simulink model "final_quadruped_070622_2"  (R2021a)
settings: Solver=VariableStepAuto  StartTime=0.0  StopTime=1  FixedStep=.001  RelTol=1e-3  EnableMultiTasking=on
undefined symbols (not defined in the file or in its folder): angleLFhip, convexoptimization, foot_x, foot_y, foot_z, height_plane, lower_leg_length, m_ll, m_ul, out, plane_x, plane_y, speedLFhip, torqueLFhip, torso_offset_x, torso_offset_z, torso_x, torso_y, torso_z, upper_leg_length, X, Y, Z
libraries: nesl_utility x151, sm_lib x71, Contact_Forces_Lib x16, fl_lib x4
(part 6 of 6)

== system final_quadruped_070622_2/Model/Right Leg Front /Knee/Subsystem ==
  In1 : Inport
  Derivative : Derivative
  Gain : Gain  Gain=100
  Gain1 : Gain  Gain=100
  Gain2 : Gain  Gain=100
  Integrator : Integrator
  Sum : Sum  Inputs=|+++
  Out1 : Outport
  wires:
  Sum/1 -> Out1/1
  Gain2/1 -> Sum/3
  In1/1 -> Derivative/1, Gain2/1, Integrator/1
  Derivative/1 -> Gain/1
  Gain/1 -> Sum/1
  Integrator/1 -> Gain1/1
  Gain1/1 -> Sum/2

== matlab function final_quadruped_070622_2/Model/Left Leg Front/Subsystem/MATLAB Function ==
  data: eb1g output; eb2g output; eb3g output; qhb input; qab input; Qquat input; qkb input; ab1g output; ab2g output; cmb1g output; cmb2g output; cmb3g output; Qd3g output
function [eb1g,eb2g,eb3g,ab1g,ab2g,cmb1g,cmb2g,cmb3g,Qd3g] = fcn(qhb,qab,Qquat,qkb)
eb1g = zeros([3 1], 'double');
eb2g = zeros([3 1], 'double');
eb3g = zeros([3 1], 'double');
ab1g = zeros([3 1], 'double');
ab2g = zeros([3 1], 'double');
cmb1g = zeros([3 1], 'double');
cmb2g = zeros([3 1], 'double');
cmb3g = zeros([3 1], 'double');
Qd3g = zeros([3 3], 'double');
coder.extrinsic('lfval_mex');
[eb1g,eb2g,eb3g,ab1g,ab2g,cmb1g,cmb2g,cmb3g,Qd3g] = lfval_mex(qhb,qab,Qquat,qkb);
end

== matlab function final_quadruped_070622_2/Model/Right Leg Back/Subsystem/MATLAB Function ==
  data: ec1g output; ec2g output; ec3g output; qhc input; qac input; Qquat input; qkc input; ac1g output; ac2g output; cmc1g output; cmc2g output; cmc3g output; Qd3g output
function [ec1g,ec2g,ec3g,ac1g,ac2g,cmc1g,cmc2g,cmc3g,Qd3g] = fcn(qhc,qac,Qquat,qkc)
ec1g = zeros([3 1], 'double');
ec2g = zeros([3 1], 'double');
ec3g = zeros([3 1], 'double');
ac1g = zeros([3 1], 'double');
ac2g = zeros([3 1], 'double');
cmc1g = zeros([3 1], 'double');
cmc2g = zeros([3 1], 'double');
cmc3g = zeros([3 1], 'double');
Qd3g = zeros([3 3], 'double');
coder.extrinsic('rbval_mex');
[ec1g,ec2g,ec3g,ac1g,ac2g,cmc1g,cmc2g,cmc3g,Qd3g] = rbval_mex(qhc,qac,Qquat,qkc);
end

== matlab function final_quadruped_070622_2/Model/Left LegBack/Subsystem/MATLAB Function ==
  data: ed1g output; ed2g output; ed3g output; qhd input; qad input; Qquat input; qkd input; ad1g output; ad2g output; cmd1g output; cmd2g output; cmd3g output; Qd3g output
function [ed1g,ed2g,ed3g,ad1g,ad2g,cmd1g,cmd2g,cmd3g,Qd3g] = fcn(qhd,qad,Qquat, qkd)
ed1g = zeros([3 1], 'double');
ed2g = zeros([3 1], 'double');
ed3g = zeros([3 1], 'double');
ad1g = zeros([3 1], 'double');
ad2g = zeros([3 1], 'double');
cmd1g = zeros([3 1], 'double');
cmd2g = zeros([3 1], 'double');
cmd3g = zeros([3 1], 'double');
Qd3g = zeros([3 3], 'double');
coder.extrinsic('lbval_mex');
[ed1g,ed2g,ed3g,ad1g,ad2g,cmd1g,cmd2g,cmd3g,Qd3g] = lbval_mex(qhd,qad,Qquat, qkd);
end

== matlab function final_quadruped_070622_2/Model/MATLAB Function4 ==
  data: hLF input; hRB input; hLB input; h_dotLF input; hRF input; h_dotRF input; tddRF output; v_torso input; tddLF output; tddRB output; tddLB output; h output; h_dot output; h_dotRB input; h_dotLB input; theta_d_des output; M output; V input
function [tddRF,tddLF,tddRB,tddLB,h,h_dot,theta_d_des,M] = fcn(hLF, hRB, hLB, h_dotLF, hRF,h_dotRF, v_torso, h_dotRB, h_dotLB, V)
% tddRF = zeros([3 1], 'double');
% tddLF = zeros([3 1], 'double');
% tddRB = zeros([3 1], 'double');
% tddLB = zeros([3 1], 'double');
% h = zeros([3 12], 'double');
% h_dot = zeros([3 12], 'double');
% theta_d_des = zeros([12 1], 'double');
% M = zeros(1, 'double');
% coder.extrinsic('theta_d_des_mex');
% [tddRF,tddLF,tddRB,tddLB,h,h_dot,theta_d_des,M] = theta_d_des_mex(hLF, hRB, hLB, h_dotLF, hRF,h_dotRF, v_torso, h_dotRB, h_dotLB);
lower_leg_length = 10;
upper_leg_length = 10;
density = 1000;
foot_density=2000;
leg_radius = 0.75;
foot_x = 8;
foot_y = 6;
foot_z = 1;
torso_y = 16;
torso_x = 25;
torso_z = 10;
m_ul=density*leg_radius*leg_radius*upper_leg_length*3.141592653589*0.01*0.01*0.01;
m_ll=density*leg_radius*leg_radius*lower_leg_length*3.141592653589*0.01*0.01*0.01;
m_foot=foot_density*foot_x*foot_y*foot_z*0.000001;
m_torso=density*torso_x*torso_y*torso_z*0.000001;
M=m_torso+(4*(m_ul+m_ll+m_foot));
%%
h=[hRF hLF hRB hLB];
% A=transpose(h)*h;
% [V,D]=eig(A);
% VR=real(V);
% %coder.extrinsic('chooseJVoptimize');
h_dot=[h_dotRF h_dotLF h_dotRB h_dotLB];
% %theta_d_des=chooseJVoptimize(h,h_dot,v_torso, M);
% % 
% theta_d_des=M*(-pinv(h)*v_torso)+VR(:,1);
% % % theta_d_des=zeros(12,1);
% % x=zeros(12,9);
% % y=zeros(12,9);
% % ynorm=zeros(9,1);
% % for i=1:9
% %     x(:,i)=M*(-pinv(h)*v_torso)+real(V(:,i));
% %     y(:,i)=pinv(h)*(-h_dot*x(:,i));
% %     ynorm(i)=norm(y(:,i));
% % end
% % ynormmin=min(ynorm);
% % 
% % for i=1:9
% %     if ynorm(i)==ynormmin
% %         theta_d_des=x(:,i);
% %     end
% % end
 w=zeros(9,1);
% %w = [0.01;0.03;0.05;0.01;0.03;0.04;0.02;0.005;0.6];
% Va=VR(:,1:9);
% %tddfun = @(w) norm(-pinv(h)*h_dot*M*(-pinv(h)*v_torso+Va*w));
% tddfun = @(w) norm(-pinv(h)*h_dot*(Va*w));
% A = Va;
% b = 0.5*ones(12,1);
% %Aeq = [transpose(x(2:10))*x(2:10)*ones(12,1),(x(1)*eye(12,12)-pinv(Reh)*Rehdot)*Va];
% Aeq = [];
% 
% beq = [];
% lb = [];
% ub =[];
% %nonlcon =norm(w)-1;
% w0 = [0.01;0.03;0.05;0.01;0.03;0.04;0.05;0.02;0.06];
% options=optimoptions('fmincon', 'Algorithm', 'sqp');
%  w= fmincon(tddfun,w0,A,b,[],[],[],[],[],options);
%theta_d_des=Va*w;
VR=real(V);
Va=VR(:,1:9);
% theta_d_des=M*(-pinv(h)*v_torso)+VR(:,1);
% Va=VR(:,1:9);
% 
% 
% w1=1;w2=2;w3=3;w4=4;w5=5;w6=6;w7=7;w8=8;w9=9;
% 
% cvx_begin
%     variables w1 w2 w3 w4 w5 w6 w7 w8 w9
%     minimize(norm(-pinv(h)*h_dot*(Va*[w1;w2;w3;w4;w5;w6;w7;w8;w9])));
%     subject to
%         Va*[w1;w2;w3;w4;w5;w6;w7;w8;w9] < 0.5*ones(12,1);
% cvx_end
% 
% w=[w1;w2;w3;w4;w5;w6;w7;w8;w9];
% theta_d_des=Va*w;

% [w]=convexoptimization(VR,h,h_dot);
 theta_d_des=Va*w;
 
tddRF_hip=theta_d_des(1);
tddRF_knee=theta_d_des(2);
tddRF_ankle=theta_d_des(3);
tddLF_hip=theta_d_des(4);
tddLF_knee=theta_d_des(5);
tddLF_ankle=theta_d_des(6);
tddRB_hip=theta_d_des(7);
tddRB_knee=theta_d_des(8);
tddRB_ankle=theta_d_des(9);
tddLB_hip=theta_d_des(10);
tddLB_knee=theta_d_des(11);
tddLB_ankle=theta_d_des(12);

tddRF=[tddRF_hip tddRF_knee tddRF_ankle];
tddLF=[tddLF_hip tddLF_knee tddLF_ankle];
tddRB=[tddRB_hip tddRB_knee tddRB_ankle];
tddLB=[tddLB_hip tddLB_knee tddLB_ankle];
end

== matlab function final_quadruped_070622_2/Model/Right Leg Front /Subsystem/MATLAB Function1 ==
  data: ea10g input; ea20g input; aa10g input; cma2 input; cma1 input; cma3 input; ea30g input; aa20g input; hRF output; rhoRF output
function [hRF,rhoRF] = fcn(ea10g, ea20g, aa10g, cma2, cma1, cma3, ea30g, aa20g)
hRF = zeros([3 3], 'double');
rhoRF = zeros([3 3 3], 'double');
coder.extrinsic('hrfrhorf_mex');
[hRF,rhoRF] = hrfrhorf_mex(ea10g, ea20g, aa10g, cma2, cma1, cma3, ea30g, aa20g);
end

== matlab function final_quadruped_070622_2/Model/Left Leg Front/Subsystem/MATLAB Function1 ==
  data: eb10g input; eb20g input; ab10g input; cmb2 input; cmb1 input; cmb3 input; eb30g input; hLF output; ab20g input; rhoLF output
function [hLF,rhoLF] = fcn(eb10g, eb20g, ab10g, cmb2, cmb1, cmb3, eb30g, ab20g)
hLF = zeros([3 3], 'double');
rhoLF = zeros([3 3 3], 'double');
coder.extrinsic('hlfrholf_mex');
[hLF,rhoLF] = hlfrholf_mex(eb10g, eb20g, ab10g, cmb2, cmb1, cmb3, eb30g, ab20g);
end

== matlab function final_quadruped_070622_2/Model/Right Leg Back/Subsystem/MATLAB Function1 ==
  data: ec10g input; ec20g input; ac10g input; cmc2 input; cmc1 input; cmc3 input; ec30g input; ac20g input; hRB output; rhoRB output
function [hRB,rhoRB] = fcn(ec10g, ec20g, ac10g, cmc2, cmc1, cmc3, ec30g, ac20g)
hRB = zeros([3 3], 'double');
rhoRB = zeros([3 3 3], 'double');
coder.extrinsic('hrbrhorb_mex');
[hRB,rhoRB] = hrbrhorb_mex(ec10g, ec20g, ac10g, cmc2, cmc1, cmc3, ec30g, ac20g);
end

== matlab function final_quadruped_070622_2/Model/Left LegBack/Subsystem/MATLAB Function1 ==
  data: ed10g input; ed20g input; ad10g input; cmd2 input; cmd1 input; cmd3 input; ed30g input; ad20g input; hLB output; rhoLB output
function [hLB,rhoLB] = fcn(ed10g, ed20g, ad10g, cmd2, cmd1, cmd3, ed30g, ad20g)
hLB = zeros([3 3], 'double');
rhoLB = zeros([3 3 3], 'double');
coder.extrinsic('hlbrholb_mex');
[hLB,rhoLB] = hlbrholb_mex(ed10g, ed20g, ad10g, cmd2, cmd1, cmd3, ed30g, ad20g);
end

== matlab function final_quadruped_070622_2/MATLAB Function ==
  data: vx input; v_torso output; vy input; vz input
function v_torso = fcn(vx, vy, vz)
v_torso=[vx; vy; vz];
end

== matlab function final_quadruped_070622_2/Model/Right Leg Front /MATLAB Function2 ==
  data: tddRF input; tddRF_hip output; tddRF_knee output; tddRF_ankle output
function [tddRF_hip, tddRF_knee, tddRF_ankle] = fcn(tddRF)
tddRF_hip = zeros(1, 'double');
tddRF_knee = zeros(1, 'double');
tddRF_ankle = zeros(1, 'double');
coder.extrinsic('rf2_mex');
[tddRF_hip, tddRF_knee, tddRF_ankle] = rf2_mex(tddRF);
end

== matlab function final_quadruped_070622_2/Subsystem/MATLAB Function1 ==
  data: vx input; vy input; v output; vz input; ax input; ay input; az input; a output
function [v,a] = fcn(vx,vy,vz,ax,ay,az)
v=[vx;vy;vz];
a=[ax;ay;az];
end

== matlab function final_quadruped_070622_2/Model/Left Leg Front/MATLAB Function2 ==
  data: tddLF input; tddLF_hip output; tddLF_knee output; tddLF_ankle output
function [tddLF_hip, tddLF_knee, tddLF_ankle] = fcn(tddLF)
tddLF_hip = zeros(1, 'double');
tddLF_knee = zeros(1, 'double');
tddLF_ankle = zeros(1, 'double');
coder.extrinsic('lf2_mex');
[tddLF_hip, tddLF_knee, tddLF_ankle] = lf2_mex(tddLF);
end

== matlab function final_quadruped_070622_2/Model/Right Leg Back/MATLAB Function2 ==
  data: tddRB input; tddRB_hip output; tddRB_knee output; tddRB_ankle output
function [tddRB_hip, tddRB_knee, tddRB_ankle] = fcn(tddRB)
tddRB_hip=zeros(1,'double');
tddRB_knee=zeros(1,'double');
tddRB_ankle=zeros(1,'double');
coder.extrinsic('rb2_mex');
[tddRB_hip, tddRB_knee, tddRB_ankle] = rb2_mex(tddRB);
end

== matlab function final_quadruped_070622_2/Model/Left LegBack/MATLAB Function2 ==
  data: tddLB input; tddLB_hip output; tddLB_knee output; tddLB_ankle output
function [tddLB_hip, tddLB_knee, tddLB_ankle] = fcn(tddLB)
tddLB_hip=zeros(1,'double');
tddLB_knee=zeros(1,'double');
tddLB_ankle=zeros(1,'double');
coder.extrinsic('lb2_mex');
[tddLB_hip, tddLB_knee, tddLB_ankle] = lb2_mex(tddLB);
end

== matlab function final_quadruped_070622_2/Subsystem/MATLAB Function4 ==
  data: vx input; vy input; v output; vz input; ax input; ay input; az input; a output
function [v,a] = fcn(vx,vy,vz,ax,ay,az)
v=[vx;vy;vz];
a=[ax;ay;az];
end

== matlab function final_quadruped_070622_2/Subsystem/MATLAB Function5 ==
  data: vx input; vy input; v output; vz input; ax input; ay input; az input; a output
function [v,a] = fcn(vx,vy,vz,ax,ay,az)
v=[vx;vy;vz];
a=[ax;ay;az];
end

== matlab function final_quadruped_070622_2/Subsystem/MATLAB Function6 ==
  data: vx input; vy input; v output; vz input; ax input; ay input; az input; a output
function [v,a] = fcn(vx,vy,vz,ax,ay,az)
v=[vx;vy;vz];
a=[ax;ay;az];
end

== matlab function final_quadruped_070622_2/Subsystem/MATLAB Function7 ==
  data: vx input; vy input; v output; vz input; ax input; ay input; az input; a output
function [v,a] = fcn(vx,vy,vz,ax,ay,az)
v=[vx;vy;vz];
a=[ax;ay;az];
end

== matlab function final_quadruped_070622_2/Subsystem/MATLAB Function8 ==
  data: vx input; vy input; v output; vz input; ax input; ay input; az input; a output
function [v,a] = fcn(vx,vy,vz,ax,ay,az)
v=[vx;vy;vz];
a=[ax;ay;az];
end

== matlab function final_quadruped_070622_2/Subsystem/MATLAB Function9 ==
  data: vx input; vy input; v output; vz input; ax input; ay input; az input; a output
function [v,a] = fcn(vx,vy,vz,ax,ay,az)
v=[vx;vy;vz];
a=[ax;ay;az];
end

== matlab function final_quadruped_070622_2/Subsystem/MATLAB Function10 ==
  data: vx input; vy input; v output; vz input; ax input; ay input; az input; a output
function [v,a] = fcn(vx,vy,vz,ax,ay,az)
v=[vx;vy;vz];
a=[ax;ay;az];
end

== matlab function final_quadruped_070622_2/Subsystem/MATLAB Function11 ==
  data: vx input; vy input; v output; vz input; ax input; ay input; az input; a output
function [v,a] = fcn(vx,vy,vz,ax,ay,az)
v=[vx;vy;vz];
a=[ax;ay;az];
end

== matlab function final_quadruped_070622_2/Subsystem/MATLAB Function13 ==
  data: vulRF input; vllRF input; Mvcm output; vfRF input; vulLF input; vllLF input; vfLF input; vulRB input; vllRB input; vfRB input; vulLB input; vllLB input; vfLB input; v_torso input; vlinks output; vcm output
function [Mvcm,vlinks,vcm] = fcn(vulRF,vllRF,vfRF,vulLF,vllLF,vfLF,vulRB,vllRB,vfRB,vulLB,vllLB,vfLB,v_torso)
%%
lower_leg_length = 10;
upper_leg_length = 10;
density = 1000;
foot_density=2000;
leg_radius = 0.75;
foot_x = 8;
foot_y = 6;
foot_z = 1;
torso_y = 16;
torso_x = 25;
torso_z = 10;
m_ul=density*leg_radius*leg_radius*upper_leg_length*3.141592653589*0.01*0.01*0.01;
m_ll=density*leg_radius*leg_radius*lower_leg_length*3.141592653589*0.01*0.01*0.01;
m_foot=foot_density*foot_x*foot_y*foot_z*0.000001;
m_torso=density*torso_x*torso_y*torso_z*0.000001;
M=m_torso+4*(m_ul+m_ll+m_foot);
%%
Mvcm=m_torso*v_torso+(m_ul*vulRF+m_ll*vllRF+m_foot*vfRF)+(m_ul*vulLF+m_ll*vllLF+m_foot*vfLF)+(m_ul*vulRB+m_ll*vllRB+m_foot*vfRB)+(m_ul*vulLB+m_ll*vllLB+m_foot*vfLB);
vlinks=[vulRF vllRF vfRF vulLF vllLF vfLF vulRB vllRB vfRB vulLB vllLB vfLB];
vcm=Mvcm/M;
end

== matlab function final_quadruped_070622_2/Subsystem/MATLAB Function12 ==
  data: vx input; vy input; v output; vz input; ax input; ay input; az input; a output
function [v,a] = fcn(vx,vy,vz,ax,ay,az)
v=[vx;vy;vz];
a=[ax;ay;az];
end

== matlab function final_quadruped_070622_2/Subsystem/MATLAB Function14 ==
  data: vx input; vy input; v output; vz input; ax input; ay input; az input; a output
function [v,a] = fcn(vx,vy,vz,ax,ay,az)
v=[vx;vy;vz];
a=[ax;ay;az];
end

== matlab function final_quadruped_070622_2/Model/Right Leg Front /MATLAB Function ==
  data: ankle input; knee input; tdRF output; hip input
function tdRF= fcn(ankle, knee, hip)
tdRF = zeros([3 1], 'double');
coder.extrinsic('rf3_mex');
tdRF=rf3_mex(ankle, knee, hip);
end

== matlab function final_quadruped_070622_2/Model/Left Leg Front/MATLAB Function ==
  data: ankle input; knee input; tdRF output; hip input
function tdRF= fcn(ankle, knee, hip)
tdRF = zeros([3 1], 'double');
coder.extrinsic('lf3_mex');
tdRF= lf3_mex(ankle, knee, hip);
end

== matlab function final_quadruped_070622_2/Model/Right Leg Back/MATLAB Function ==
  data: ankle input; knee input; tdRB output; hip input
function tdRB= fcn(ankle, knee, hip)
tdRB=zeros([3 1],'double');
coder.extrinsic('rb3_mex');
tdRB= rb3_mex(ankle, knee, hip);
end

== matlab function final_quadruped_070622_2/Model/Left LegBack/MATLAB Function ==
  data: ankle input; knee input; tdLB output; hip input
function tdLB= fcn(ankle, knee, hip)
tdLB=zeros([3 1],'double');
coder.extrinsic('lb3_mex');
tdLB= lb3_mex(ankle, knee, hip);
end

== matlab function final_quadruped_070622_2/Model/MATLAB Function ==
  data: tdRF input; td output; tdLF input; tdRB input; tdLB input; t2dRF input; t2dLF input; t2dRB input; t2dLB input; t2d output
function [td,t2d] = fcn(tdRF,tdLF,tdRB,tdLB,t2dRF,t2dLF,t2dRB,t2dLB)
td = zeros([12 1], 'double');
t2d = zeros([12 1], 'double');
coder.extrinsic('acttheta_mex');
[td,t2d] = acttheta_mex(tdRF,tdLF,tdRB,tdLB,t2dRF,t2dLF,t2dRB,t2dLB);
end

== matlab function final_quadruped_070622_2/Model/MATLAB Function1 ==
  data: h input; h_dot input; ht2d output; td input; t2d input; h_dottd output; htd output; theta_d_des input; theta_2d_des input; ht2ddes output; hdtddes output
function [ht2d,h_dottd,htd,ht2ddes,hdtddes] = fcn(h,h_dot, td, t2d,theta_d_des,theta_2d_des)
ht2d = zeros([3 1], 'double');
h_dottd = zeros([3 1], 'double');
htd = zeros([3 1], 'double');
ht2ddes = zeros([3 1], 'double');
hdtddes = zeros([3 1], 'double');
coder.extrinsic('findh_mex');
[ht2d,h_dottd,htd,ht2ddes,hdtddes] = findh_mex(h,h_dot, td, t2d,theta_d_des,theta_2d_des);
end

== matlab function final_quadruped_070622_2/MATLAB Function1 ==
  data: Mvcm input; error output; ht2d input; h_dottd input; a_torso input; v_torso input; f input; Macm input; htd input; ht2ddes input; hdtddes input
function error = fcn(Mvcm,ht2d,h_dottd,a_torso, v_torso, f,Macm,htd, ht2ddes, hdtddes)
%%
lower_leg_length = 10;
upper_leg_length = 10;
density = 1000;
foot_density=2000;
leg_radius = 0.75;
foot_x = 8;
foot_y = 6;
foot_z = 1;
torso_y = 16;
torso_x = 25;
torso_z = 10;
m_ul=density*leg_radius*leg_radius*upper_leg_length*3.141592653589*0.01*0.01*0.01;
m_ll=density*leg_radius*leg_radius*lower_leg_length*3.141592653589*0.01*0.01*0.01;
m_foot=foot_density*foot_x*foot_y*foot_z*0.000001;
m_torso=density*torso_x*torso_y*torso_z*0.000001;
M=m_torso+(4*(m_ul+m_ll+m_foot));
g=[0; 0; -9.80067];
%%
error1=htd+M*v_torso-Mvcm;
error2=ht2d+h_dottd+M*a_torso-M*g-f-Macm;
error=ht2ddes+hdtddes+M*a_torso-M*g-f-Macm;
end

== matlab function final_quadruped_070622_2/Model/Right Leg Front /Subsystem/MATLAB Function2 ==
  data: h_dotRF output; ea_dg1 input; ea1g input; ea2g input; ea3g input; ea_dg2 input; ea_dg3 input; rho_dotRF input; rhoRF input
function h_dotRF = fcn(  ea_dg1,ea1g, ea2g, ea3g, ea_dg2, ea_dg3, rho_dotRF, rhoRF)
h_dotRF = zeros([3 3], 'double');
coder.extrinsic('hdotrf_mex');
h_dotRF = hdotrf_mex(ea_dg1,ea1g, ea2g, ea3g, ea_dg2, ea_dg3, rho_dotRF, rhoRF);
end

== matlab function final_quadruped_070622_2/Model/Left Leg Front/Subsystem/MATLAB Function2 ==
  data: h_dotLF output; eb_dg1 input; eb1g input; eb2g input; eb3g input; eb_dg2 input; eb_dg3 input; rho_dotLF input; rhoLF input
function h_dotLF = fcn( eb_dg1,eb1g, eb2g, eb3g, eb_dg2, eb_dg3, rho_dotLF, rhoLF)
h_dotLF = zeros([3 3], 'double');
coder.extrinsic('hdotlf_mex');
h_dotLF = hdotlf_mex( eb_dg1,eb1g, eb2g, eb3g, eb_dg2, eb_dg3, rho_dotLF, rhoLF);

end

== matlab function final_quadruped_070622_2/Model/Right Leg Front /Subsystem/MATLAB Function4 ==
  data: ea1g input; ea2g input; aa1g input; aa2g input; ea3g input; vlinks input; w_torso input; ea_dg1 output; td1 input; v_torso input; ea_dg2 output; td2 input; td3 input; ea_dg3 output; rho_dotRF output
function [ea_dg1,ea_dg2,ea_dg3,rho_dotRF] = fcn(ea1g,ea2g,aa1g,aa2g, ea3g, vlinks, w_torso, td1, v_torso, td2, td3)
ea_dg1 = zeros([3 1], 'double');
ea_dg2 = zeros([3 1], 'double');
ea_dg3 = zeros([3 1], 'double');
rho_dotRF = zeros([3 3 3], 'double');
coder.extrinsic('rfval1_mex');
[ea_dg1,ea_dg2,ea_dg3,rho_dotRF] = rfval1_mex(ea1g,ea2g,aa1g,aa2g, ea3g, vlinks, w_torso, td1, v_torso, td2, td3);

end

== matlab function final_quadruped_070622_2/Model/Left Leg Front/Subsystem/MATLAB Function4 ==
  data: eb1g input; eb2g input; ab1g input; ab2g input; eb3g input; vlinks input; w_torso input; eb_dg1 output; td1 input; v_torso input; eb_dg2 output; td2 input; td3 input; eb_dg3 output; rho_dotLF output
function [eb_dg1,eb_dg2,eb_dg3,rho_dotLF] = fcn(eb1g,eb2g,ab1g,ab2g, eb3g, vlinks, w_torso, td1, v_torso, td2, td3)
eb_dg1 = zeros([3 1], 'double');
eb_dg2 = zeros([3 1], 'double');
eb_dg3 = zeros([3 1], 'double');
rho_dotLF = zeros([3 3 3], 'double');
coder.extrinsic('lfval1_mex');
[eb_dg1,eb_dg2,eb_dg3,rho_dotLF] = lfval1_mex(eb1g,eb2g,ab1g,ab2g, eb3g, vlinks, w_torso, td1, v_torso, td2, td3);

end

== matlab function final_quadruped_070622_2/Model/Right Leg Back/Subsystem/MATLAB Function2 ==
  data: h_dotRB output; ec_dg1 input; ec1g input; ec2g input; ec3g input; ec_dg2 input; ec_dg3 input; rho_dotRB input; rhoRB input
function h_dotRB = fcn( ec_dg1,ec1g, ec2g, ec3g, ec_dg2, ec_dg3, rho_dotRB, rhoRB)
h_dotRB = zeros([3 3], 'double');
coder.extrinsic('hdotrb_mex');
h_dotRB = hdotrb_mex( ec_dg1,ec1g, ec2g, ec3g, ec_dg2, ec_dg3, rho_dotRB, rhoRB);
end

== matlab function final_quadruped_070622_2/Model/Right Leg Back/Subsystem/MATLAB Function4 ==
  data: ec1g input; ec2g input; ac1g input; ac2g input; ec3g input; vlinks input; w_torso input; ec_dg1 output; td1 input; v_torso input; ec_dg2 output; td2 input; td3 input; ec_dg3 output; rho_dotRB output
function [ec_dg1,ec_dg2,ec_dg3,rho_dotRB] = fcn(ec1g,ec2g,ac1g,ac2g, ec3g, vlinks, w_torso, td1, v_torso, td2, td3)
ec_dg1 = zeros([3 1], 'double');
ec_dg2 = zeros([3 1], 'double');
ec_dg3 = zeros([3 1], 'double');
rho_dotRB = zeros([3 3 3], 'double');
coder.extrinsic('rbval1_mex');
[ec_dg1,ec_dg2,ec_dg3,rho_dotRB] = rbval1_mex(ec1g,ec2g,ac1g,ac2g, ec3g, vlinks, w_torso, td1, v_torso, td2, td3);

end

== matlab function final_quadruped_070622_2/Subsystem/MATLAB Function2 ==
  data: vx input; vy input; v output; vz input; ax input; ay input; az input; a output
function [v,a] = fcn(vx,vy,vz,ax,ay,az)
v=[vx;vy;vz];
a=[ax;ay;az];
end

== matlab function final_quadruped_070622_2/Model/Left LegBack/Subsystem/MATLAB Function2 ==
  data: h_dotLB output; ed_dg1 input; ed1g input; ed2g input; ed3g input; ed_dg2 input; ed_dg3 input; rho_dotLB input; rhoLB input
function h_dotLB = fcn( ed_dg1,ed1g, ed2g, ed3g, ed_dg2, ed_dg3, rho_dotLB, rhoLB)
h_dotLB = zeros([3 3], 'double');
coder.extrinsic('hdotlb_mex');
h_dotLB = hdotlb_mex( ed_dg1,ed1g, ed2g, ed3g, ed_dg2, ed_dg3, rho_dotLB, rhoLB);
end

== matlab function final_quadruped_070622_2/Model/Left LegBack/Subsystem/MATLAB Function4 ==
  data: ed1g input; ed2g input; ad1g input; ad2g input; ed3g input; vlinks input; w_torso input; ed_dg1 output; td1 input; v_torso input; ed_dg2 output; td2 input; td3 input; ed_dg3 output; rho_dotLB output
function [ed_dg1,ed_dg2,ed_dg3,rho_dotLB] = fcn(ed1g,ed2g,ad1g,ad2g, ed3g, vlinks, w_torso, td1, v_torso, td2, td3)
ed_dg1 = zeros([3 1], 'double');
ed_dg2 = zeros([3 1], 'double');
ed_dg3 = zeros([3 1], 'double');
rho_dotLB = zeros([3 3 3], 'double');
coder.extrinsic('lbval1_mex');
[ed_dg1,ed_dg2,ed_dg3,rho_dotLB] = lbval1_mex(ed1g,ed2g,ad1g,ad2g, ed3g, vlinks, w_torso, td1, v_torso, td2, td3);
end

== matlab function final_quadruped_070622_2/Model/Left Leg Front/MATLAB Function1 ==
  data: ankle input; knee input; t2dLF output; hip input
function t2dLF= fcn(ankle, knee, hip)
t2dLF = zeros([3 1], 'double');
coder.extrinsic('lf4_mex');
t2dLF= lf4_mex(ankle, knee, hip);
end

== matlab function final_quadruped_070622_2/Model/Right Leg Front /MATLAB Function1 ==
  data: ankle input; knee input; t2dRF output; hip input
function t2dRF= fcn(ankle, knee, hip)
t2dRF = zeros([3 1], 'double');
coder.extrinsic('rf4_mex');
t2dRF= rf4_mex(ankle, knee, hip);
end

== matlab function final_quadruped_070622_2/MATLAB Function2 ==
  data: ax input; a_torso output; ay input; az input
function a_torso = fcn(ax, ay, az)
a_torso=[ax; ay; az];
end

== matlab function final_quadruped_070622_2/Model/Left Leg Front/Contact Forces /MATLAB Function ==
  data: n1 input; NLF output; n2 input; n4 input; n3 input; f1 input; f2 input; f3 input; f4 input; FLF output; Qd3g input
function [NLF,FLF] = fcn(n1,n2,n4,n3,f1,f2,f3,f4, Qd3g)
Qds3=[1 0 0;
      0 cos(90) -sin(90);
      0 sin(90) cos(90)];
% mu_s = 0.8;
% alpha=atan(mu_s);
% NRF=n1+n2+n3+n4;
% FRFca=f1*cos(alpha)+f2*cos(alpha)+f3*cos(alpha)+f4*cos(alpha);
% FRFsa=f1*sin(alpha)+f2*sin(alpha)+f3*sin(alpha)+f4*sin(alpha);
NLF=n1+n2+n3+n4;
FLF=f1+f2+f3+f4;
FLF=Qds3*Qd3g*FLF;
end

== matlab function final_quadruped_070622_2/Model/MATLAB Function2 ==
  data: theta_d_des input; theta_2d_des output; h_dot input; h input; a_torso input; M input; f input
function theta_2d_des = fcn(theta_d_des, h_dot, h, a_torso, M, f)
 theta_2d_des = zeros([12 1], 'double');
 coder.extrinsic('theta_2d_des_mex'); 
 theta_2d_des=theta_2d_des_mex(theta_d_des, h_dot, h, a_torso, M, f);
%theta_2d_des=zeros([12 1],'double');
end

== matlab function final_quadruped_070622_2/Model/Right Leg Front /Contact Forces /MATLAB Function ==
  data: n1 input; NRF output; n2 input; n4 input; n3 input; f1 input; f2 input; f3 input; f4 input; FRF output; Qd3g input
function [NRF,FRF] = fcn(n1,n2,n4,n3,f1,f2,f3,f4, Qd3g)
% mu_s = 0.8;
% alpha=atan(mu_s);
% NRF=n1+n2+n3+n4;
% FRFca=f1*cos(alpha)+f2*cos(alpha)+f3*cos(alpha)+f4*cos(alpha);
% FRFsa=f1*sin(alpha)+f2*sin(alpha)+f3*sin(alpha)+f4*sin(alpha);
Qds3=[1 0 0;
      0 cos(90) -sin(90);
      0 sin(90) cos(90)];
NRF=n1+n2+n3+n4;
FRFl=f1+f2+f3+f4;
FRF=Qds3*Qd3g*FRFl;
end

== matlab function final_quadruped_070622_2/Model/Right Leg Back/Contact Forces /MATLAB Function ==
  data: n1 input; NRB output; n2 input; n4 input; n3 input; f1 input; f2 input; f3 input; f4 input; FRB output; Qd3g input
function [NRB,FRB] = fcn(n1,n2,n4,n3,f1,f2,f3,f4,Qd3g)
Qds3=[1 0 0;
      0 cos(90) -sin(90);
      0 sin(90) cos(90)];
% mu_s = 0.8;
% alpha=atan(mu_s);
% NRF=n1+n2+n3+n4;
% FRFca=f1*cos(alpha)+f2*cos(alpha)+f3*cos(alpha)+f4*cos(alpha);
% FRFsa=f1*sin(alpha)+f2*sin(alpha)+f3*sin(alpha)+f4*sin(alpha);
NRB=n1+n2+n3+n4;
FRB=f1+f2+f3+f4;
FRB=Qds3*Qd3g*FRB;
end

== matlab function final_quadruped_070622_2/Subsystem/MATLAB Function3 ==
  data: vx input; vy input; v output; vz input; ax input; ay input; az input; a output
function [v,a] = fcn(vx,vy,vz,ax,ay,az)
v=[vx;vy;vz];
a=[ax;ay;az];
end

== matlab function final_quadruped_070622_2/Model/Left LegBack/Contact Forces /MATLAB Function ==
  data: n1 input; NLB output; n2 input; n4 input; n3 input; f1 input; f2 input; f3 input; f4 input; FLB output; Qd3g input
function [NLB,FLB] = fcn(n1,n2,n4,n3,f1,f2,f3,f4, Qd3g)
Qds3=[1 0 0;
      0 cos(90) -sin(90);
      0 sin(90) cos(90)];
% mu_s = 0.8;
% alpha=atan(mu_s);
% NRF=n1+n2+n3+n4;
% FRFca=f1*cos(alpha)+f2*cos(alpha)+f3*cos(alpha)+f4*cos(alpha);
% FRFsa=f1*sin(alpha)+f2*sin(alpha)+f3*sin(alpha)+f4*sin(alpha);
NLB=n1+n2+n3+n4;
FLB=f1+f2+f3+f4;
FLB=Qds3*Qd3g*FLB;
end

== matlab function final_quadruped_070622_2/Model/MATLAB Function3 ==
  data: NRF input; f output; FRF input; NLF input; FLF input; NRB input; FRB input; NLB input; FLB input
function f = fcn(NRF,FRF,NLF,FLF,NRB,FRB, NLB,FLB)
N=NRF+NLF+NRB+NLB;
F=FRF+FLF+FRB+FLB;
f=[-F(1);-F(2); N+F(3)];
end

== matlab function final_quadruped_070622_2/Model/Right Leg Front /MATLAB Function3 ==
  data: theta_2d_des input; t2ddhip output; t2ddknee output; t2ddankle output
function [t2ddhip,t2ddknee,t2ddankle] = fcn(theta_2d_des)
t2ddhip = zeros(1, 'double');
t2ddknee = zeros(1, 'double');
t2ddankle = zeros(1, 'double');
coder.extrinsic('rf1_mex');

[t2ddhip,t2ddknee,t2ddankle] = rf1_mex(theta_2d_des);
end

== matlab function final_quadruped_070622_2/Model/Left Leg Front/MATLAB Function3 ==
  data: theta_2d_des input; t2ddhip output; t2ddknee output; t2ddankle output
function [t2ddhip,t2ddknee,t2ddankle] = fcn(theta_2d_des)
t2ddhip = zeros(1, 'double');
t2ddknee = zeros(1, 'double');
t2ddankle = zeros(1, 'double');
coder.extrinsic('lf1_mex');
[t2ddhip,t2ddknee,t2ddankle] = lf1_mex(theta_2d_des);
end

== matlab function final_quadruped_070622_2/Model/Right Leg Back/MATLAB Function3 ==
  data: theta_2d_des input; t2ddhip output; t2ddknee output; t2ddankle output
function [t2ddhip,t2ddknee,t2ddankle] = fcn(theta_2d_des)
t2ddhip=zeros(1,'double');
t2ddknee=zeros(1,'double');
t2ddankle=zeros(1,'double');
coder.extrinsic('rb1_mex');

[t2ddhip,t2ddknee,t2ddankle] = rb1_mex(theta_2d_des);
end

== matlab function final_quadruped_070622_2/Model/Left LegBack/MATLAB Function3 ==
  data: theta_2d_des input; t2ddhip output; t2ddknee output; t2ddankle output
function [t2ddhip,t2ddknee,t2ddankle] = fcn(theta_2d_des)
t2ddhip=zeros(1,'double');
t2ddknee=zeros(1,'double');
t2ddankle=zeros(1,'double');
coder.extrinsic('lb1_mex');
[t2ddhip,t2ddknee,t2ddankle] = lb1_mex(theta_2d_des);
end

== matlab function final_quadruped_070622_2/Model/Right Leg Back/MATLAB Function1 ==
  data: ankle input; knee input; t2dRB output; hip input
function t2dRB= fcn(ankle, knee, hip)
t2dRB=zeros([3 1],'double');
coder.extrinsic('rb4_mex');
t2dRB= rb4_mex(ankle, knee, hip);
end

== matlab function final_quadruped_070622_2/Model/Left LegBack/MATLAB Function1 ==
  data: ankle input; knee input; t2dLB output; hip input
function t2dLB= fcn(ankle, knee, hip)
t2dLB=zeros([3 1],'double');
coder.extrinsic('lb4_mex');
t2dLB= lb4_mex(ankle, knee, hip);
end

== matlab function final_quadruped_070622_2/Subsystem/MATLAB Function ==
  data: aulRF input; Macm output; allRF input; afRF input; aulLF input; allLF input; afLF input; aulRB input; allRB input; afRB input; aulLB input; allLB input; afLB input; a_torso input; alinks output; acm output
function [Macm,alinks,acm] = fcn(aulRF,allRF,afRF,aulLF,allLF,afLF,aulRB,allRB,afRB,aulLB,allLB,afLB,a_torso)
%%
lower_leg_length = 10;
upper_leg_length = 10;
density = 1000;
foot_density=2000;
leg_radius = 0.75;
foot_x = 8;
foot_y = 6;
foot_z = 1;
torso_y = 16;
torso_x = 25;
torso_z = 10;
m_ul=density*leg_radius*leg_radius*upper_leg_length*3.141592653589*0.01*0.01*0.01;
m_ll=density*leg_radius*leg_radius*lower_leg_length*3.141592653589*0.01*0.01*0.01;
m_foot=foot_density*foot_x*foot_y*foot_z*0.000001;
m_torso=density*torso_x*torso_y*torso_z*0.000001;
M=m_torso+4*(m_ul+m_ll+m_foot);
%%
Macm=m_torso*a_torso+(m_ul*aulRF+m_ll*allRF+m_foot*afRF)+(m_ul*aulLF+m_ll*allLF+m_foot*afLF)+(m_ul*aulRB+m_ll*allRB+m_foot*afRB)+(m_ul*aulLB+m_ll*allLB+m_foot*afLB);
alinks=[aulRF allRF afRF aulLF allLF afLF aulRB allRB afRB aulLB allLB afLB];
acm=Macm/M;
end

== matlab function final_quadruped_070622_2/Model/MATLAB Function5 ==
  data: hLF input; h output; hRB input; hLB input; h_dotLF input; hRF input; h_dotRF input; h_dotRB input; h_dotLB input; h_dot output
function [h,h_dot] = fcn(hLF, hRB, hLB, h_dotLF, hRF,h_dotRF,h_dotRB,h_dotLB)
h=[hRF hLF hRB hLB];
h_dot=[h_dotRF h_dotLF h_dotRB h_dotLB];
end

== matlab function final_quadruped_070622_2/Model/MATLAB Function6 ==
  data: out output; h input; h_dot input; V output
function [out,V] = fcn(h,h_dot)
A=transpose(h)*h;
% V=eye(12,12);
% D=eye(12,12);
[V,D]=eig(A);
V=real(V);
out = [h;h_dot;V];
end

== matlab function final_quadruped_070622_2/Model/Right Leg Front /Subsystem/MATLAB Function ==
  data: ea1g output; ea2g output; ea3g output; qha input; qaa input; Qquat input; qka input; aa1g output; aa2g output; cma1g output; cma2g output; cma3g output; Qd3g output
function [ea1g,ea2g,ea3g,aa1g,aa2g,cma1g,cma2g,cma3g,Qd3g] = fcn(qha,qaa,Qquat,qka)
ea1g = zeros([3 1], 'double');
ea2g = zeros([3 1], 'double');
ea3g = zeros([3 1], 'double');
aa1g = zeros([3 1], 'double');
aa2g = zeros([3 1], 'double');
cma1g = zeros([3 1], 'double');
cma2g = zeros([3 1], 'double');
cma3g = zeros([3 1], 'double');
Qd3g = zeros([3 3], 'double');
coder.extrinsic('rfval_mex');
[ea1g,ea2g,ea3g,aa1g,aa2g,cma1g,cma2g,cma3g,Qd3g] = rfval_mex(qha,qaa,Qquat,qka);

end
